simulink model "lecture8_heatex"  (Simulink 7.1)
settings: Solver=FixedStepDiscrete  StartTime=0.0  StopTime=10.0  RelTol=1e-3
settings Model: Creator=pit  LastModifiedBy=pit

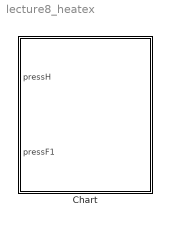
== system lecture8_heatex ==
  Chart : Stateflow chart

== stateflow chart Chart ==
  state Off
  state H
  state F
  (default) -> Off
  Off -> H [order 1] : [pressH=1]
  H -> Off [order 2] : [pressH=0]
  H -> F [order 1] : [pressF=1]
  F -> H [order 1] : [pressH=1]
  Off -> F [order 2] : [pressF=1]
  F -> Off [order 2] : [pressF=0]
  data: pressH input double; pressF1 input double
